simulink library "halout"  (R2021b)
settings: Solver=VariableStepAuto  StartTime=0.0  StopTime=10.0  RelTol=1e-3
undefined symbols (not defined in the file): C_TASK_5MS_S, FALSE, KHAL_CAN1FD1APS3E2E_flg, KHAL_CAN1FD1APS3TxReq_flg, KHAL_CAN1FD1VCU2E2E_flg, KHAL_CAN1FD1VCU2TxReq_flg, KHAL_CAN1FD1VCU3E2E_flg, KHAL_CAN1FD1VCU3TxReq_flg, KHAL_CAN1TxReq_flg, KHAL_CAN1VMCFCM1E2E_flg, KHAL_CAN1VMCFCM1TxReq_flg, KHAL_CAN2TxReq_flg, KHAL_CAN3FD3VCU1toNIDECTxReq_flg, KHAL_CAN3FD3VCU1TxReq_flg, KHAL_CAN3FD3VCU2E2E_flg, KHAL_CAN3FD3VCU2toNIDECE2E_flg, KHAL_CAN3FD3VCU2toNIDECTxReq_flg, KHAL_CAN3FD3VCU2TxReq_flg, KHAL_CAN3TxReq_flg, KHAL_CAN4FD4CE1000E2E_flg, KHAL_CAN4FD4CE1000TxReq_flg, KHAL_CAN4TxReq_flg, KHAL_CAN5TxReq_flg, KHAL_CAN6FD6APS3E2E_flg, KHAL_CAN6FD6APS3TxReq_flg, KHAL_CAN6FD6VCU2E2E_flg, KHAL_CAN6FD6VCU2TxReq_flg, KHAL_CAN6TxReq_flg, ONE_INT, TRUE, ZERO_INT
libraries: FVT_lib x551, simulink x244
(part 25 of 26)

== system halout/HAL_OUT/CAN6/FD6_VCU2_0x154/Byte_11 ==
  VehActPwr : Inport
  BitwiseOR : simulink/Logic and Bit Operations/Bitwise Operator  logicop=OR  UseBitMask=off  BitMask=bin2dec('11011001')  BitMaskRealWorld=Stored Integer
  SignalPack : FVT_lib/hal/SignalPack  RightShiftCnt=8  BitMask=2^8-1  LeftShiftCnt=0
  UnitConverter : DataTypeConversion  OutDataTypeStr=uint8  RndMeth=Round
  UnitConverter1 : DataTypeConversion  OutDataTypeStr=uint32  RndMeth=Round
  convert_out : FVT_lib/hal/convert_out  gain=1  offset=-600000
  Byte_11 : Outport
  wires:
  BitwiseOR/1 -> Byte_11/1
  UnitConverter/1 -> BitwiseOR/1
  SignalPack/1 -> UnitConverter/1
  UnitConverter1/1 -> SignalPack/1
  convert_out/1 -> UnitConverter1/1
  VehActPwr/1 -> convert_out/1

== system halout/HAL_OUT/CAN6/FD6_VCU2_0x154/Byte_12 ==
  VehActPwr : Inport
  BitwiseOR : simulink/Logic and Bit Operations/Bitwise Operator  logicop=OR  UseBitMask=off  BitMask=bin2dec('11011001')  BitMaskRealWorld=Stored Integer
  SignalPack : FVT_lib/hal/SignalPack  RightShiftCnt=0  BitMask=2^8-1  LeftShiftCnt=0
  UnitConverter : DataTypeConversion  OutDataTypeStr=uint8  RndMeth=Round
  UnitConverter1 : DataTypeConversion  OutDataTypeStr=uint32  RndMeth=Round
  convert_out : FVT_lib/hal/convert_out  gain=1  offset=-600000
  Byte_12 : Outport
  wires:
  BitwiseOR/1 -> Byte_12/1
  UnitConverter/1 -> BitwiseOR/1
  SignalPack/1 -> UnitConverter/1
  UnitConverter1/1 -> SignalPack/1
  convert_out/1 -> UnitConverter1/1
  VehActPwr/1 -> convert_out/1

== system halout/HAL_OUT/CAN6/FD6_VCU2_0x154/Byte_13 ==
  DriverTq : Inport
  BitwiseOR : simulink/Logic and Bit Operations/Bitwise Operator  logicop=OR  UseBitMask=off  BitMask=bin2dec('11011001')  BitMaskRealWorld=Stored Integer
  SignalPack : FVT_lib/hal/SignalPack  RightShiftCnt=8  BitMask=2^8-1  LeftShiftCnt=0
  UnitConverter : DataTypeConversion  OutDataTypeStr=uint8  RndMeth=Round
  UnitConverter1 : DataTypeConversion  OutDataTypeStr=uint16  RndMeth=Round
  convert_out : FVT_lib/hal/convert_out  gain=1  offset=-4300
  Byte_13 : Outport
  wires:
  BitwiseOR/1 -> Byte_13/1
  UnitConverter/1 -> BitwiseOR/1
  SignalPack/1 -> UnitConverter/1
  UnitConverter1/1 -> SignalPack/1
  convert_out/1 -> UnitConverter1/1
  DriverTq/1 -> convert_out/1

== system halout/HAL_OUT/CAN6/FD6_VCU2_0x154/Byte_14 ==
  DriverTq : Inport
  BitwiseOR : simulink/Logic and Bit Operations/Bitwise Operator  logicop=OR  UseBitMask=off  BitMask=bin2dec('11011001')  BitMaskRealWorld=Stored Integer
  SignalPack : FVT_lib/hal/SignalPack  RightShiftCnt=0  BitMask=2^8-1  LeftShiftCnt=0
  UnitConverter : DataTypeConversion  OutDataTypeStr=uint8  RndMeth=Round
  UnitConverter1 : DataTypeConversion  OutDataTypeStr=uint16  RndMeth=Round
  convert_out : FVT_lib/hal/convert_out  gain=1  offset=-4300
  Byte_14 : Outport
  wires:
  BitwiseOR/1 -> Byte_14/1
  UnitConverter/1 -> BitwiseOR/1
  SignalPack/1 -> UnitConverter/1
  UnitConverter1/1 -> SignalPack/1
  convert_out/1 -> UnitConverter1/1
  DriverTq/1 -> convert_out/1

== system halout/HAL_OUT/CAN6/FD6_VCU2_0x154/Byte_15 ==
  ActAPSPosn : Inport
  BitwiseOR : simulink/Logic and Bit Operations/Bitwise Operator  logicop=OR  UseBitMask=off  BitMask=bin2dec('11011001')  BitMaskRealWorld=Stored Integer
  SignalPack : FVT_lib/hal/SignalPack  RightShiftCnt=0  BitMask=2^8-1  LeftShiftCnt=0
  UnitConverter : DataTypeConversion  OutDataTypeStr=uint8  RndMeth=Round
  UnitConverter1 : DataTypeConversion  OutDataTypeStr=uint8  RndMeth=Round
  convert_out : FVT_lib/hal/convert_out  gain=0.394  offset=0
  Byte_15 : Outport
  wires:
  BitwiseOR/1 -> Byte_15/1
  UnitConverter/1 -> BitwiseOR/1
  SignalPack/1 -> UnitConverter/1
  UnitConverter1/1 -> SignalPack/1
  convert_out/1 -> UnitConverter1/1
  ActAPSPosn/1 -> convert_out/1

== system halout/HAL_OUT/CAN6/FD6_VCU2_0x154/Byte_2 ==
  Fr_DriverTq : Inport
  BitwiseOR : simulink/Logic and Bit Operations/Bitwise Operator  logicop=OR  UseBitMask=off  BitMask=bin2dec('11011001')  BitMaskRealWorld=Stored Integer
  SignalPack : FVT_lib/hal/SignalPack  RightShiftCnt=8  BitMask=2^8-1  LeftShiftCnt=0
  UnitConverter : DataTypeConversion  OutDataTypeStr=uint8  RndMeth=Round
  UnitConverter1 : DataTypeConversion  OutDataTypeStr=uint16  RndMeth=Round
  convert_out : FVT_lib/hal/convert_out  gain=0.5  offset=-5300
  Byte_2 : Outport
  wires:
  BitwiseOR/1 -> Byte_2/1
  UnitConverter/1 -> BitwiseOR/1
  SignalPack/1 -> UnitConverter/1
  UnitConverter1/1 -> SignalPack/1
  convert_out/1 -> UnitConverter1/1
  Fr_DriverTq/1 -> convert_out/1

== system halout/HAL_OUT/CAN6/FD6_VCU2_0x154/Byte_3 ==
  Fr_DriverTq : Inport
  BitwiseOR : simulink/Logic and Bit Operations/Bitwise Operator  logicop=OR  UseBitMask=off  BitMask=bin2dec('11011001')  BitMaskRealWorld=Stored Integer
  SignalPack : FVT_lib/hal/SignalPack  RightShiftCnt=0  BitMask=2^8-1  LeftShiftCnt=0
  UnitConverter : DataTypeConversion  OutDataTypeStr=uint8  RndMeth=Round
  UnitConverter1 : DataTypeConversion  OutDataTypeStr=uint16  RndMeth=Round
  convert_out : FVT_lib/hal/convert_out  gain=0.5  offset=-5300
  Byte_3 : Outport
  wires:
  BitwiseOR/1 -> Byte_3/1
  UnitConverter/1 -> BitwiseOR/1
  SignalPack/1 -> UnitConverter/1
  UnitConverter1/1 -> SignalPack/1
  convert_out/1 -> UnitConverter1/1
  Fr_DriverTq/1 -> convert_out/1

== system halout/HAL_OUT/CAN6/FD6_VCU2_0x154/Byte_4 ==
  Rr_DriverTq : Inport
  BitwiseOR : simulink/Logic and Bit Operations/Bitwise Operator  logicop=OR  UseBitMask=off  BitMask=bin2dec('11011001')  BitMaskRealWorld=Stored Integer
  SignalPack : FVT_lib/hal/SignalPack  RightShiftCnt=8  BitMask=2^8-1  LeftShiftCnt=0
  UnitConverter : DataTypeConversion  OutDataTypeStr=uint8  RndMeth=Round
  UnitConverter1 : DataTypeConversion  OutDataTypeStr=uint16  RndMeth=Round
  convert_out : FVT_lib/hal/convert_out  gain=0.5  offset=-5300
  Byte_4 : Outport
  wires:
  BitwiseOR/1 -> Byte_4/1
  UnitConverter/1 -> BitwiseOR/1
  SignalPack/1 -> UnitConverter/1
  UnitConverter1/1 -> SignalPack/1
  convert_out/1 -> UnitConverter1/1
  Rr_DriverTq/1 -> convert_out/1

== system halout/HAL_OUT/CAN6/FD6_VCU2_0x154/Byte_5 ==
  Rr_DriverTq : Inport
  BitwiseOR : simulink/Logic and Bit Operations/Bitwise Operator  logicop=OR  UseBitMask=off  BitMask=bin2dec('11011001')  BitMaskRealWorld=Stored Integer
  SignalPack : FVT_lib/hal/SignalPack  RightShiftCnt=0  BitMask=2^8-1  LeftShiftCnt=0
  UnitConverter : DataTypeConversion  OutDataTypeStr=uint8  RndMeth=Round
  UnitConverter1 : DataTypeConversion  OutDataTypeStr=uint16  RndMeth=Round
  convert_out : FVT_lib/hal/convert_out  gain=0.5  offset=-5300
  Byte_5 : Outport
  wires:
  BitwiseOR/1 -> Byte_5/1
  UnitConverter/1 -> BitwiseOR/1
  SignalPack/1 -> UnitConverter/1
  UnitConverter1/1 -> SignalPack/1
  convert_out/1 -> UnitConverter1/1
  Rr_DriverTq/1 -> convert_out/1

== system halout/HAL_OUT/CAN6/FD6_VCU2_0x154/Byte_6 ==
  ACC_CtrlAvail : Inport
  AccPedal_Override : Inport  Port=2
  BitwiseOR : simulink/Logic and Bit Operations/Bitwise Operator  logicop=OR  UseBitMask=off  NumInputPorts=2  BitMask=bin2dec('11011001')  BitMaskRealWorld=Stored Integer
  SignalPack : FVT_lib/hal/SignalPack  RightShiftCnt=0  BitMask=2^1-1  LeftShiftCnt=7
  SignalPack1 : FVT_lib/hal/SignalPack  RightShiftCnt=0  BitMask=2^1-1  LeftShiftCnt=6
  UnitConverter{,1..3} (4 alike) : DataTypeConversion  OutDataTypeStr=uint8  RndMeth=Round
  Byte_6 : Outport
  wires:
  BitwiseOR/1 -> Byte_6/1
  UnitConverter/1 -> BitwiseOR/1
  SignalPack/1 -> UnitConverter/1
  UnitConverter1/1 -> SignalPack/1
  ACC_CtrlAvail/1 -> UnitConverter1/1
  UnitConverter2/1 -> BitwiseOR/2
  SignalPack1/1 -> UnitConverter2/1
  UnitConverter3/1 -> SignalPack1/1
  AccPedal_Override/1 -> UnitConverter3/1

== system halout/HAL_OUT/CAN6/FD6_VCU2_0x154/CRC8_IfAction_Tx ==
  CAN_E2E_flg : Inport
  DataID1 : Inport  Port=2
  DataID2 : Inport  Port=3
  RawData : Inport  Port=4
  Data Type Conversion : DataTypeConversion  OutDataTypeStr=uint8
  If : If
  If Action Subsystem : Subsystem  TreatAsAtomicUnit=on
  If Action Subsystem1 : Subsystem  TreatAsAtomicUnit=on
  Merge : Merge
  CRC8 : Outport
  wires:
  If/2 -> If Action Subsystem/Action
  If/1 -> If Action Subsystem1/Action
  CAN_E2E_flg/1 -> [CAN_E2E_flg]
  DataID1/1 -> [DataID1]
  DataID2/1 -> [DataID2]
  RawData/1 -> [RawData]
  [CAN_E2E_flg] -> Data Type Conversion/1
  [DataID1] -> If Action Subsystem1/1(CAN_E2E_ID1)
  [DataID2] -> If Action Subsystem1/2(CAN_E2E_ID2)
  [RawData] -> If Action Subsystem1/3(Byte1)
  [RawData] -> If Action Subsystem/1(Byte1)
  If Action Subsystem1/1(CRC8_E2EResult) -> Merge/1
  If Action Subsystem/1(CRC8_Result) -> Merge/2
  Merge/1 -> CRC8/1
  Data Type Conversion/1 -> If/1

== system halout/HAL_OUT/CAN6/FD6_VCU2_0x154/CSVCU2CAN6 ==
  CSVCU2CAN6 : Inport
  Data Type Conversion : DataTypeConversion  OutDataTypeStr=uint8  RndMeth=Round
  CAN6_CS_VCU2_CAN6 : Outport
  wires:
  Data Type Conversion/1 -> CAN6_CS_VCU2_CAN6/1
  CSVCU2CAN6/1 -> Data Type Conversion/1

== system halout/HAL_OUT/CAN6/FD6_VCU2_0x154/DriverTq ==
  DriverTq : Inport
  Data Type Conversion : DataTypeConversion  OutDataTypeStr=uint16  RndMeth=Round
  convert_out : FVT_lib/hal/convert_out  gain=1  offset=-4300
  CAN6_DriverTq : Outport
  wires:
  Data Type Conversion/1 -> CAN6_DriverTq/1
  convert_out/1 -> Data Type Conversion/1
  DriverTq/1 -> convert_out/1

== system halout/HAL_OUT/CAN6/FD6_VCU2_0x154/FrDriverTq ==
  FrDriverTq : Inport
  Data Type Conversion : DataTypeConversion  OutDataTypeStr=uint16  RndMeth=Round
  convert_out : FVT_lib/hal/convert_out  gain=0.5  offset=-5300
  CAN6_Fr_DriverTq : Outport
  wires:
  Data Type Conversion/1 -> CAN6_Fr_DriverTq/1
  convert_out/1 -> Data Type Conversion/1
  FrDriverTq/1 -> convert_out/1

== system halout/HAL_OUT/CAN6/FD6_VCU2_0x154/RCVCU2CAN6 ==
  RCVCU2CAN6 : Inport
  Data Type Conversion : DataTypeConversion  OutDataTypeStr=uint8  RndMeth=Round
  CAN6_RC_VCU2_CAN6 : Outport
  wires:
  Data Type Conversion/1 -> CAN6_RC_VCU2_CAN6/1
  RCVCU2CAN6/1 -> Data Type Conversion/1

== system halout/HAL_OUT/CAN6/FD6_VCU2_0x154/RrDriverTq ==
  RrDriverTq : Inport
  Data Type Conversion : DataTypeConversion  OutDataTypeStr=uint16  RndMeth=Round
  convert_out : FVT_lib/hal/convert_out  gain=0.5  offset=-5300
  CAN6_Rr_DriverTq : Outport
  wires:
  Data Type Conversion/1 -> CAN6_Rr_DriverTq/1
  convert_out/1 -> Data Type Conversion/1
  RrDriverTq/1 -> convert_out/1

== system halout/HAL_OUT/CAN6/FD6_VCU2_0x154/VehActPwr ==
  VehActPwr : Inport
  Data Type Conversion : DataTypeConversion  OutDataTypeStr=uint32  RndMeth=Round
  convert_out : FVT_lib/hal/convert_out  gain=1  offset=-600000
  CAN6_VehActPwr : Outport
  wires:
  Data Type Conversion/1 -> CAN6_VehActPwr/1
  convert_out/1 -> Data Type Conversion/1
  VehActPwr/1 -> convert_out/1

== system halout/HAL_OUT/CAN6/FD6_VMC1_0x17F/AccCalcuPID ==
  AccCalcuPID : Inport
  Data Type Conversion : DataTypeConversion  OutDataTypeStr=uint16  RndMeth=Round
  convert_out : FVT_lib/hal/convert_out  gain=0.05  offset=-15
  CAN6_AccCalcuPID : Outport
  wires:
  Data Type Conversion/1 -> CAN6_AccCalcuPID/1
  convert_out/1 -> Data Type Conversion/1
  AccCalcuPID/1 -> convert_out/1

== system halout/HAL_OUT/CAN6/FD6_VMC1_0x17F/CCMSASpdWar ==
  CCMSASpdWar : Inport
  Data Type Conversion : DataTypeConversion  OutDataTypeStr=uint8  RndMeth=Round
  CAN6_CCMSA_SpdWar : Outport
  wires:
  Data Type Conversion/1 -> CAN6_CCMSA_SpdWar/1
  CCMSASpdWar/1 -> Data Type Conversion/1

== system halout/HAL_OUT/CAN6/FD6_VMC1_0x17F/DISCButtSta ==
  DISCButtSta : Inport
  Data Type Conversion : DataTypeConversion  OutDataTypeStr=uint8  RndMeth=Round
  CAN6_DISC_ButtSta : Outport
  wires:
  Data Type Conversion/1 -> CAN6_DISC_ButtSta/1
  DISCButtSta/1 -> Data Type Conversion/1

== system halout/HAL_OUT/CAN6/FD6_VMC1_0x17F/DISCDISCTargetSpd ==
  DISCDISCTargetSpd : Inport
  Data Type Conversion : DataTypeConversion  OutDataTypeStr=uint16  RndMeth=Round
  convert_out : FVT_lib/hal/convert_out  gain=0.125  offset=0
  CAN6_DISC_DISCTargetSpd : Outport
  wires:
  Data Type Conversion/1 -> CAN6_DISC_DISCTargetSpd/1
  convert_out/1 -> Data Type Conversion/1
  DISCDISCTargetSpd/1 -> convert_out/1

== system halout/HAL_OUT/CAN6/FD6_VMC1_0x17F/DISCDISCTurn ==
  DISCDISCTurn : Inport
  Data Type Conversion : DataTypeConversion  OutDataTypeStr=uint8  RndMeth=Round
  CAN6_DISC_DISCTurn : Outport
  wires:
  Data Type Conversion/1 -> CAN6_DISC_DISCTurn/1
  DISCDISCTurn/1 -> Data Type Conversion/1

== system halout/HAL_OUT/CAN6/FD6_VMC1_0x17F/DISCReqAcc ==
  DISCReqAcc : Inport
  Data Type Conversion : DataTypeConversion  OutDataTypeStr=uint16  RndMeth=Round
  convert_out : FVT_lib/hal/convert_out  gain=0.05  offset=-15
  CAN6_DISCReqAcc : Outport
  wires:
  Data Type Conversion/1 -> CAN6_DISCReqAcc/1
  convert_out/1 -> Data Type Conversion/1
  DISCReqAcc/1 -> convert_out/1

== system halout/HAL_OUT/CAN6/FD6_VMC1_0x17F/DISCSta ==
  DISCSta : Inport
  Data Type Conversion : DataTypeConversion  OutDataTypeStr=uint8  RndMeth=Round
  CAN6_DISC_Sta : Outport
  wires:
  Data Type Conversion/1 -> CAN6_DISC_Sta/1
  DISCSta/1 -> Data Type Conversion/1

== system halout/HAL_OUT/CAN6/FD6_VMC1_0x17F/FDCVMCLongAccelCmd ==
  FDCVMCLongAccelCmd : Inport
  Data Type Conversion : DataTypeConversion  OutDataTypeStr=uint8  RndMeth=Round
  convert_out : FVT_lib/hal/convert_out  gain=0.01  offset=-1.27
  CAN6_FDC_VMC_LongAccel_Cmd : Outport
  wires:
  Data Type Conversion/1 -> CAN6_FDC_VMC_LongAccel_Cmd/1
  convert_out/1 -> Data Type Conversion/1
  FDCVMCLongAccelCmd/1 -> convert_out/1

== system halout/HAL_OUT/CAN6/FD6_VMC1_0x17F/FeatArbitrFinal ==
  FeatArbitrFinal : Inport
  Data Type Conversion : DataTypeConversion  OutDataTypeStr=uint8  RndMeth=Round
  CAN6_FeatArbitrFinal : Outport
  wires:
  Data Type Conversion/1 -> CAN6_FeatArbitrFinal/1
  FeatArbitrFinal/1 -> Data Type Conversion/1

== system halout/HAL_OUT/CAN6/FD6_VMC1_0x17F/FeatArbitrSta ==
  FeatArbitrSta : Inport
  Data Type Conversion : DataTypeConversion  OutDataTypeStr=uint8  RndMeth=Round
  CAN6_FeatArbitrSta : Outport
  wires:
  Data Type Conversion/1 -> CAN6_FeatArbitrSta/1
  FeatArbitrSta/1 -> Data Type Conversion/1

== system halout/HAL_OUT/CAN6/FD6_VMC1_0x17F/FeatReqSpd ==
  FeatReqSpd : Inport
  Data Type Conversion : DataTypeConversion  OutDataTypeStr=uint16  RndMeth=Round
  convert_out : FVT_lib/hal/convert_out  gain=0.125  offset=0
  CAN6_FeatReqSpd : Outport
  wires:
  Data Type Conversion/1 -> CAN6_FeatReqSpd/1
  convert_out/1 -> Data Type Conversion/1
  FeatReqSpd/1 -> convert_out/1

== system halout/HAL_OUT/CAN6/FD6_VMC1_0x17F/FeatSetSpdFinalraw32 ==
  FeatSetSpdFinalraw32 : Inport
  Data Type Conversion : DataTypeConversion  OutDataTypeStr=uint8  RndMeth=Round
  CAN6_FeatSetSpdFinal_raw32 : Outport
  wires:
  Data Type Conversion/1 -> CAN6_FeatSetSpdFinal_raw32/1
  FeatSetSpdFinalraw32/1 -> Data Type Conversion/1

== system halout/HAL_OUT/CAN6/FD6_VMC1_0x17F/FrontRearSlipRatioCtrl ==
  FrontRearSlipRatioCtrl : Inport
  Data Type Conversion : DataTypeConversion  OutDataTypeStr=uint8  RndMeth=Round
  CAN6_FrontRearSlipRatioCtrl : Outport
  wires:
  Data Type Conversion/1 -> CAN6_FrontRearSlipRatioCtrl/1
  FrontRearSlipRatioCtrl/1 -> Data Type Conversion/1

== system halout/HAL_OUT/CAN6/FD6_VMC1_0x17F/JerkPCT ==
  JerkPCT : Inport
  Data Type Conversion : DataTypeConversion  OutDataTypeStr=uint8  RndMeth=Round
  CAN6_JerkPCT : Outport
  wires:
  Data Type Conversion/1 -> CAN6_JerkPCT/1
  JerkPCT/1 -> Data Type Conversion/1

== system halout/HAL_OUT/CAN6/FD6_VMC1_0x17F/LatAccCtrl ==
  LatAccCtrl : Inport
  Data Type Conversion : DataTypeConversion  OutDataTypeStr=uint8  RndMeth=Round
  CAN6_LatAccCtrl : Outport
  wires:
  Data Type Conversion/1 -> CAN6_LatAccCtrl/1
  LatAccCtrl/1 -> Data Type Conversion/1

== system halout/HAL_OUT/CAN6/FD6_VMC1_0x17F/LateralCtrl ==
  LateralCtrl : Inport
  Data Type Conversion : DataTypeConversion  OutDataTypeStr=uint8  RndMeth=Round
  CAN6_LateralCtrl : Outport
  wires:
  Data Type Conversion/1 -> CAN6_LateralCtrl/1
  LateralCtrl/1 -> Data Type Conversion/1

== system halout/HAL_OUT/CAN6/FD6_VMC1_0x17F/LimitPCT ==
  LimitPCT : Inport
  Data Type Conversion : DataTypeConversion  OutDataTypeStr=uint8  RndMeth=Round
  CAN6_LimitPCT : Outport
  wires:
  Data Type Conversion/1 -> CAN6_LimitPCT/1
  LimitPCT/1 -> Data Type Conversion/1

== system halout/HAL_OUT/CAN6/FD6_VMC1_0x17F/MeterIndSpeedraw32 ==
  MeterIndSpeedraw32 : Inport
  Data Type Conversion : DataTypeConversion  OutDataTypeStr=uint8  RndMeth=Round
  CAN6_MeterIndSpeed_raw32 : Outport
  wires:
  Data Type Conversion/1 -> CAN6_MeterIndSpeed_raw32/1
  MeterIndSpeedraw32/1 -> Data Type Conversion/1

== system halout/HAL_OUT/CAN6/FD6_VMC1_0x17F/RearWhlSlipRatioCtrl ==
  RearWhlSlipRatioCtrl : Inport
  Data Type Conversion : DataTypeConversion  OutDataTypeStr=uint8  RndMeth=Round
  CAN6_RearWhlSlipRatioCtrl : Outport
  wires:
  Data Type Conversion/1 -> CAN6_RearWhlSlipRatioCtrl/1
  RearWhlSlipRatioCtrl/1 -> Data Type Conversion/1

== system halout/HAL_OUT/CAN6/FD6_VMC1_0x17F/SPD2ACCAct ==
  SPD2ACCAct : Inport
  Data Type Conversion : DataTypeConversion  OutDataTypeStr=uint8  RndMeth=Round
  CAN6_SPD2ACCAct : Outport
  wires:
  Data Type Conversion/1 -> CAN6_SPD2ACCAct/1
  SPD2ACCAct/1 -> Data Type Conversion/1

== system halout/HAL_OUT/CAN6/FD6_VMC1_0x17F/SafetyCtrl ==
  SafetyCtrl : Inport
  Data Type Conversion : DataTypeConversion  OutDataTypeStr=uint8  RndMeth=Round
  CAN6_SafetyCtrl : Outport
  wires:
  Data Type Conversion/1 -> CAN6_SafetyCtrl/1
  SafetyCtrl/1 -> Data Type Conversion/1

== system halout/HAL_OUT/CAN6/FD6_VMC1_0x17F/SingleWhlSlipRatioCtrl ==
  SingleWhlSlipRatioCtrl : Inport
  Data Type Conversion : DataTypeConversion  OutDataTypeStr=uint8  RndMeth=Round
  CAN6_SingleWhlSlipRatioCtrl : Outport
  wires:
  Data Type Conversion/1 -> CAN6_SingleWhlSlipRatioCtrl/1
  SingleWhlSlipRatioCtrl/1 -> Data Type Conversion/1

== system halout/HAL_OUT/CAN6/FD6_VMC1_0x17F/TimeGapCalcu ==
  TimeGapCalcu : Inport
  Data Type Conversion : DataTypeConversion  OutDataTypeStr=uint8  RndMeth=Round
  convert_out : FVT_lib/hal/convert_out  gain=0.1  offset=0
  CAN6_TimeGapCalcu : Outport
  wires:
  Data Type Conversion/1 -> CAN6_TimeGapCalcu/1
  convert_out/1 -> Data Type Conversion/1
  TimeGapCalcu/1 -> convert_out/1

== system halout/HAL_OUT/CAN6/FD6_VMC1_0x17F/VMCACCCtrlAvail ==
  VMCACCCtrlAvail : Inport
  Data Type Conversion : DataTypeConversion  OutDataTypeStr=uint8  RndMeth=Round
  CAN6_VMC_ACCCtrlAvail : Outport
  wires:
  Data Type Conversion/1 -> CAN6_VMC_ACCCtrlAvail/1
  VMCACCCtrlAvail/1 -> Data Type Conversion/1

== system halout/HAL_OUT/CAN6/FD6_VMC1_0x17F/VMCAEBCtrlAvail ==
  VMCAEBCtrlAvail : Inport
  Data Type Conversion : DataTypeConversion  OutDataTypeStr=uint8  RndMeth=Round
  CAN6_VMC_AEBCtrlAvail : Outport
  wires:
  Data Type Conversion/1 -> CAN6_VMC_AEBCtrlAvail/1
  VMCAEBCtrlAvail/1 -> Data Type Conversion/1

== system halout/HAL_OUT/CAN6/FD6_VMC1_0x17F/VMCCCCtrlAvail ==
  VMCCCCtrlAvail : Inport
  Data Type Conversion : DataTypeConversion  OutDataTypeStr=uint8  RndMeth=Round
  CAN6_VMC_CCCtrlAvail : Outport
  wires:
  Data Type Conversion/1 -> CAN6_VMC_CCCtrlAvail/1
  VMCCCCtrlAvail/1 -> Data Type Conversion/1

== system halout/HAL_OUT/CAN6/FD6_VMC1_0x17F/VMCMSACtrlAvail ==
  VMCMSACtrlAvail : Inport
  Data Type Conversion : DataTypeConversion  OutDataTypeStr=uint8  RndMeth=Round
  CAN6_VMC_MSACtrlAvail : Outport
  wires:
  Data Type Conversion/1 -> CAN6_VMC_MSACtrlAvail/1
  VMCMSACtrlAvail/1 -> Data Type Conversion/1

== system halout/HAL_OUT/CAN6/FD6_VMC1_0x17F/VMCVCUACCCtrlAvail ==
  VMCVCUACCCtrlAvail : Inport
  Data Type Conversion : DataTypeConversion  OutDataTypeStr=uint8  RndMeth=Round
  CAN6_VMC_VCU_ACC_CtrlAvail : Outport
  wires:
  Data Type Conversion/1 -> CAN6_VMC_VCU_ACC_CtrlAvail/1
  VMCVCUACCCtrlAvail/1 -> Data Type Conversion/1

== system halout/HAL_OUT/CAN6/FD6_VMC1_0x17F/VMCVCUAPSCtrlAvailflg ==
  VMCVCUAPSCtrlAvailflg : Inport
  Data Type Conversion : DataTypeConversion  OutDataTypeStr=uint8  RndMeth=Round
  CAN6_VMC_VCU_APSCtrlAvail_flg : Outport
  wires:
  Data Type Conversion/1 -> CAN6_VMC_VCU_APSCtrlAvail_flg/1
  VMCVCUAPSCtrlAvailflg/1 -> Data Type Conversion/1

== system halout/HAL_OUT/CAN6/FD6_VMC1_0x17F/VMCVCUAccPedalOverride ==
  VMCVCUAccPedalOverride : Inport
  Data Type Conversion : DataTypeConversion  OutDataTypeStr=uint8  RndMeth=Round
  CAN6_VMC_VCU_AccPedal_Override : Outport
  wires:
  Data Type Conversion/1 -> CAN6_VMC_VCU_AccPedal_Override/1
  VMCVCUAccPedalOverride/1 -> Data Type Conversion/1

== system halout/HAL_OUT/CAN6/FD6_VMC1_0x17F/VMCVCUCCCrlSta ==
  VMCVCUCCCrlSta : Inport
  Data Type Conversion : DataTypeConversion  OutDataTypeStr=uint8  RndMeth=Round
  CAN6_VMC_VCU_CC_Crl_Sta : Outport
  wires:
  Data Type Conversion/1 -> CAN6_VMC_VCU_CC_Crl_Sta/1
  VMCVCUCCCrlSta/1 -> Data Type Conversion/1

== system halout/HAL_OUT/CAN6/FD6_VMC1_0x17F/VMCVCUMSACrlSta ==
  VMCVCUMSACrlSta : Inport
  Data Type Conversion : DataTypeConversion  OutDataTypeStr=uint8  RndMeth=Round
  CAN6_VMC_VCU_MSA_Crl_Sta : Outport
  wires:
  Data Type Conversion/1 -> CAN6_VMC_VCU_MSA_Crl_Sta/1
  VMCVCUMSACrlSta/1 -> Data Type Conversion/1

== system halout/HAL_OUT/CAN6/FD6_VMC1_0x17F/VehicleSpeedkph ==
  VehicleSpeedkph : Inport
  Data Type Conversion : DataTypeConversion  OutDataTypeStr=uint16  RndMeth=Round
  convert_out : FVT_lib/hal/convert_out  gain=0.125  offset=0
  CAN6_VehicleSpeed_kph : Outport
  wires:
  Data Type Conversion/1 -> CAN6_VehicleSpeed_kph/1
  convert_out/1 -> Data Type Conversion/1
  VehicleSpeedkph/1 -> convert_out/1

== system halout/HAL_OUT/CAN6/FD6_VMC1_0x17F/VehicleSpeedmph ==
  VehicleSpeedmph : Inport
  Data Type Conversion : DataTypeConversion  OutDataTypeStr=uint16  RndMeth=Round
  convert_out : FVT_lib/hal/convert_out  gain=0.125  offset=0
  CAN6_VehicleSpeed_mph : Outport
  wires:
  Data Type Conversion/1 -> CAN6_VehicleSpeed_mph/1
  convert_out/1 -> Data Type Conversion/1
  VehicleSpeedmph/1 -> convert_out/1

== system halout/HAL_OUT/CAN6/GW6_CE100_0_0x1C6/FDCBCMDimSw ==
  FDCBCMDimSw : Inport
  Data Type Conversion : DataTypeConversion  OutDataTypeStr=uint8  RndMeth=Round
  CAN6_FDC_BCM_DimSw : Outport
  wires:
  Data Type Conversion/1 -> CAN6_FDC_BCM_DimSw/1
  FDCBCMDimSw/1 -> Data Type Conversion/1

== system halout/HAL_OUT/CAN6/GW6_CE100_0_0x1C6/FDCBCMFWipSwSta ==
  FDCBCMFWipSwSta : Inport
  Data Type Conversion : DataTypeConversion  OutDataTypeStr=uint8  RndMeth=Round
  CAN6_FDC_BCM_FWipSw_Sta : Outport
  wires:
  Data Type Conversion/1 -> CAN6_FDC_BCM_FWipSw_Sta/1
  FDCBCMFWipSwSta/1 -> Data Type Conversion/1

== system halout/HAL_OUT/CAN6/GW6_CE100_0_0x1C6/FDCBCMLLeftStaCmd ==
  FDCBCMLLeftStaCmd : Inport
  Data Type Conversion : DataTypeConversion  OutDataTypeStr=uint8  RndMeth=Round
  CAN6_FDC_BCM_LLeftSta_Cmd : Outport
  wires:
  Data Type Conversion/1 -> CAN6_FDC_BCM_LLeftSta_Cmd/1
  FDCBCMLLeftStaCmd/1 -> Data Type Conversion/1

== system halout/HAL_OUT/CAN6/GW6_CE100_0_0x1C6/FDCBCMLRightStaCmd ==
  FDCBCMLRightStaCmd : Inport
  Data Type Conversion : DataTypeConversion  OutDataTypeStr=uint8  RndMeth=Round
  CAN6_FDC_BCM_LRightSta_Cmd : Outport
  wires:
  Data Type Conversion/1 -> CAN6_FDC_BCM_LRightSta_Cmd/1
  FDCBCMLRightStaCmd/1 -> Data Type Conversion/1

== system halout/HAL_OUT/CAN6/GW6_CE100_0_0x1C6/FDCBCMPassSWSta ==
  FDCBCMPassSWSta : Inport
  Data Type Conversion : DataTypeConversion  OutDataTypeStr=uint8  RndMeth=Round
  CAN6_FDC_BCM_PassSW_Sta : Outport
  wires:
  Data Type Conversion/1 -> CAN6_FDC_BCM_PassSW_Sta/1
  FDCBCMPassSWSta/1 -> Data Type Conversion/1

== system halout/HAL_OUT/CAN6/GW6_CE100_0_0x1C6/FDCBCMTurnSwSta ==
  FDCBCMTurnSwSta : Inport
  Data Type Conversion : DataTypeConversion  OutDataTypeStr=uint8  RndMeth=Round
  CAN6_FDC_BCM_TurnSw_Sta : Outport
  wires:
  Data Type Conversion/1 -> CAN6_FDC_BCM_TurnSw_Sta/1
  FDCBCMTurnSwSta/1 -> Data Type Conversion/1

== system halout/HAL_OUT/CAN6/GW6_CE100_0_0x1C6/FDCVMCSpdCtrlModeSta ==
  FDCVMCSpdCtrlModeSta : Inport
  Data Type Conversion : DataTypeConversion  OutDataTypeStr=uint8  RndMeth=Round
  CAN6_FDC_VMC_SpdCtrlMode_Sta : Outport
  wires:
  Data Type Conversion/1 -> CAN6_FDC_VMC_SpdCtrlMode_Sta/1
  FDCVMCSpdCtrlModeSta/1 -> Data Type Conversion/1

== system halout/HAL_OUT/CAN6/GW6_CE100_0_0x1C6/FDCVMCSpdCtrlSta ==
  FDCVMCSpdCtrlSta : Inport
  Data Type Conversion : DataTypeConversion  OutDataTypeStr=uint8  RndMeth=Round
  CAN6_FDC_VMC_SpdCtrl_Sta : Outport
  wires:
  Data Type Conversion/1 -> CAN6_FDC_VMC_SpdCtrl_Sta/1
  FDCVMCSpdCtrlSta/1 -> Data Type Conversion/1

== system halout/HAL_OUT/CAN1/FD1_APS3_0x238/CRC8_IfAction_Tx/If Action Subsystem ==
  Byte1 : Inport
  Action Port : ActionPort
  CRC8_Caculation : Subsystem
      mask help: MeasumentTrigerEvent
      mask Display: fprintf('CRC8');
  CRC8_Result : Outport
  wires:
  CRC8_Caculation/1(CRCout) -> CRC8_Result/1
  Byte1/1 -> CRC8_Caculation/1(MsgData)

== system halout/HAL_OUT/CAN1/FD1_APS3_0x238/CRC8_IfAction_Tx/If Action Subsystem1 ==
  CAN_E2E_ID1 : Inport
  CAN_E2E_ID2 : Inport  Port=2
  Byte1 : Inport  Port=3
  Action Port : ActionPort
  CRC8_E2EProfile1 : Subsystem
      mask help: MeasumentTrigerEvent
      mask Display: fprintf('CRC8_E2EProfile1');
  Mux2 : Mux  Inputs=3
  CRC8_E2EResult : Outport
  wires:
  Mux2/1 -> CRC8_E2EProfile1/1(MsgData)
  CAN_E2E_ID1/1 -> Mux2/1
  CAN_E2E_ID2/1 -> Mux2/2
  Byte1/1 -> Mux2/3
  CRC8_E2EProfile1/1(CRCout) -> CRC8_E2EResult/1

== system halout/HAL_OUT/CAN1/FD1_VCU2_0x154/CRC8_IfAction_Tx/If Action Subsystem ==
  Byte1 : Inport
  Action Port : ActionPort
  CRC8_Caculation : Subsystem
      mask help: MeasumentTrigerEvent
      mask Display: fprintf('CRC8');
  CRC8_Result : Outport
  wires:
  CRC8_Caculation/1(CRCout) -> CRC8_Result/1
  Byte1/1 -> CRC8_Caculation/1(MsgData)

== system halout/HAL_OUT/CAN1/FD1_VCU2_0x154/CRC8_IfAction_Tx/If Action Subsystem1 ==
  CAN_E2E_ID1 : Inport
  CAN_E2E_ID2 : Inport  Port=2
  Byte1 : Inport  Port=3
  Action Port : ActionPort
  CRC8_E2EProfile1 : Subsystem
      mask help: MeasumentTrigerEvent
      mask Display: fprintf('CRC8_E2EProfile1');
  Mux2 : Mux  Inputs=3
  CRC8_E2EResult : Outport
  wires:
  Mux2/1 -> CRC8_E2EProfile1/1(MsgData)
  CAN_E2E_ID1/1 -> Mux2/1
  CAN_E2E_ID2/1 -> Mux2/2
  Byte1/1 -> Mux2/3
  CRC8_E2EProfile1/1(CRCout) -> CRC8_E2EResult/1

== system halout/HAL_OUT/CAN1/FD1_VCU3_0x159/CRC8_IfAction_Tx/If Action Subsystem ==
  Byte1 : Inport
  Action Port : ActionPort
  CRC8_Caculation : Subsystem
      mask help: MeasumentTrigerEvent
      mask Display: fprintf('CRC8');
  CRC8_Result : Outport
  wires:
  CRC8_Caculation/1(CRCout) -> CRC8_Result/1
  Byte1/1 -> CRC8_Caculation/1(MsgData)

== system halout/HAL_OUT/CAN1/FD1_VCU3_0x159/CRC8_IfAction_Tx/If Action Subsystem1 ==
  CAN_E2E_ID1 : Inport
  CAN_E2E_ID2 : Inport  Port=2
  Byte1 : Inport  Port=3
  Action Port : ActionPort
  CRC8_E2EProfile1 : Subsystem
      mask help: MeasumentTrigerEvent
      mask Display: fprintf('CRC8_E2EProfile1');
  Mux2 : Mux  Inputs=3
  CRC8_E2EResult : Outport
  wires:
  Mux2/1 -> CRC8_E2EProfile1/1(MsgData)
  CAN_E2E_ID1/1 -> Mux2/1
  CAN_E2E_ID2/1 -> Mux2/2
  Byte1/1 -> Mux2/3
  CRC8_E2EProfile1/1(CRCout) -> CRC8_E2EResult/1

== system halout/HAL_OUT/CAN1/VMC_FCM1_0x172/CRC8_IfAction_Tx/If Action Subsystem ==
  Byte1 : Inport
  Action Port : ActionPort
  CRC8_Caculation : Subsystem
      mask help: MeasumentTrigerEvent
      mask Display: fprintf('CRC8');
  CRC8_Result : Outport
  wires:
  CRC8_Caculation/1(CRCout) -> CRC8_Result/1
  Byte1/1 -> CRC8_Caculation/1(MsgData)

== system halout/HAL_OUT/CAN1/VMC_FCM1_0x172/CRC8_IfAction_Tx/If Action Subsystem1 ==
  CAN_E2E_ID1 : Inport
  CAN_E2E_ID2 : Inport  Port=2
  Byte1 : Inport  Port=3
  Action Port : ActionPort
  CRC8_E2EProfile1 : Subsystem
      mask help: MeasumentTrigerEvent
      mask Display: fprintf('CRC8_E2EProfile1');
  Mux2 : Mux  Inputs=3
  CRC8_E2EResult : Outport
  wires:
  Mux2/1 -> CRC8_E2EProfile1/1(MsgData)
  CAN_E2E_ID1/1 -> Mux2/1
  CAN_E2E_ID2/1 -> Mux2/2
  Byte1/1 -> Mux2/3
  CRC8_E2EProfile1/1(CRCout) -> CRC8_E2EResult/1

== system halout/HAL_OUT/CAN3/FD3_VCU2_0x153/CRC8_IfAction_Tx/If Action Subsystem ==
  Byte1 : Inport
  Action Port : ActionPort
  CRC8_Caculation : Subsystem
      mask help: MeasumentTrigerEvent
      mask Display: fprintf('CRC8');
  CRC8_Result : Outport
  wires:
  CRC8_Caculation/1(CRCout) -> CRC8_Result/1
  Byte1/1 -> CRC8_Caculation/1(MsgData)

== system halout/HAL_OUT/CAN3/FD3_VCU2_0x153/CRC8_IfAction_Tx/If Action Subsystem1 ==
  CAN_E2E_ID1 : Inport
  CAN_E2E_ID2 : Inport  Port=2
  Byte1 : Inport  Port=3
  Action Port : ActionPort
  CRC8_E2EProfile1 : Subsystem
      mask help: MeasumentTrigerEvent
      mask Display: fprintf('CRC8_E2EProfile1');
  Mux2 : Mux  Inputs=3
  CRC8_E2EResult : Outport
  wires:
  Mux2/1 -> CRC8_E2EProfile1/1(MsgData)
  CAN_E2E_ID1/1 -> Mux2/1
  CAN_E2E_ID2/1 -> Mux2/2
  Byte1/1 -> Mux2/3
  CRC8_E2EProfile1/1(CRCout) -> CRC8_E2EResult/1

== system halout/HAL_OUT/CAN3/FD3_VCU2_toNIDEC_0x154/CRC8_IfAction_Tx/If Action Subsystem ==
  Byte1 : Inport
  Action Port : ActionPort
  CRC8_Caculation : Subsystem
      mask help: MeasumentTrigerEvent
      mask Display: fprintf('CRC8');
  CRC8_Result : Outport
  wires:
  CRC8_Caculation/1(CRCout) -> CRC8_Result/1
  Byte1/1 -> CRC8_Caculation/1(MsgData)

== system halout/HAL_OUT/CAN3/FD3_VCU2_toNIDEC_0x154/CRC8_IfAction_Tx/If Action Subsystem1 ==
  CAN_E2E_ID1 : Inport
  CAN_E2E_ID2 : Inport  Port=2
  Byte1 : Inport  Port=3
  Action Port : ActionPort
  CRC8_E2EProfile1 : Subsystem
      mask help: MeasumentTrigerEvent
      mask Display: fprintf('CRC8_E2EProfile1');
  Mux2 : Mux  Inputs=3
  CRC8_E2EResult : Outport
  wires:
  Mux2/1 -> CRC8_E2EProfile1/1(MsgData)
  CAN_E2E_ID1/1 -> Mux2/1
  CAN_E2E_ID2/1 -> Mux2/2
  Byte1/1 -> Mux2/3
  CRC8_E2EProfile1/1(CRCout) -> CRC8_E2EResult/1

== system halout/HAL_OUT/CAN4/FD4_CE100_0_0x116/CRC8_IfAction_Tx/If Action Subsystem ==
  Byte1 : Inport
  Action Port : ActionPort
  CRC8_Caculation : Subsystem
      mask help: MeasumentTrigerEvent
      mask Display: fprintf('CRC8');
  CRC8_Result : Outport
  wires:
  CRC8_Caculation/1(CRCout) -> CRC8_Result/1
  Byte1/1 -> CRC8_Caculation/1(MsgData)

== system halout/HAL_OUT/CAN4/FD4_CE100_0_0x116/CRC8_IfAction_Tx/If Action Subsystem1 ==
  CAN_E2E_ID1 : Inport
  CAN_E2E_ID2 : Inport  Port=2
  Byte1 : Inport  Port=3
  Action Port : ActionPort
  CRC8_E2EProfile1 : Subsystem
      mask help: MeasumentTrigerEvent
      mask Display: fprintf('CRC8_E2EProfile1');
  Mux2 : Mux  Inputs=3
  CRC8_E2EResult : Outport
  wires:
  Mux2/1 -> CRC8_E2EProfile1/1(MsgData)
  CAN_E2E_ID1/1 -> Mux2/1
  CAN_E2E_ID2/1 -> Mux2/2
  Byte1/1 -> Mux2/3
  CRC8_E2EProfile1/1(CRCout) -> CRC8_E2EResult/1

== system halout/HAL_OUT/CAN6/FD6_APS3_0x238/CRC8_IfAction_Tx/If Action Subsystem ==
  Byte1 : Inport
  Action Port : ActionPort
  CRC8_Caculation : Subsystem
      mask help: MeasumentTrigerEvent
      mask Display: fprintf('CRC8');
  CRC8_Result : Outport
  wires:
  CRC8_Caculation/1(CRCout) -> CRC8_Result/1
  Byte1/1 -> CRC8_Caculation/1(MsgData)

== system halout/HAL_OUT/CAN6/FD6_APS3_0x238/CRC8_IfAction_Tx/If Action Subsystem1 ==
  CAN_E2E_ID1 : Inport
  CAN_E2E_ID2 : Inport  Port=2
  Byte1 : Inport  Port=3
  Action Port : ActionPort
  CRC8_E2EProfile1 : Subsystem
      mask help: MeasumentTrigerEvent
      mask Display: fprintf('CRC8_E2EProfile1');
  Mux2 : Mux  Inputs=3
  CRC8_E2EResult : Outport
  wires:
  Mux2/1 -> CRC8_E2EProfile1/1(MsgData)
  CAN_E2E_ID1/1 -> Mux2/1
  CAN_E2E_ID2/1 -> Mux2/2
  Byte1/1 -> Mux2/3
  CRC8_E2EProfile1/1(CRCout) -> CRC8_E2EResult/1

== system halout/HAL_OUT/CAN6/FD6_VCU2_0x154/CRC8_IfAction_Tx/If Action Subsystem ==
  Byte1 : Inport
  Action Port : ActionPort
  CRC8_Caculation : Subsystem
      mask help: MeasumentTrigerEvent
      mask Display: fprintf('CRC8');
  CRC8_Result : Outport
  wires:
  CRC8_Caculation/1(CRCout) -> CRC8_Result/1
  Byte1/1 -> CRC8_Caculation/1(MsgData)

== system halout/HAL_OUT/CAN6/FD6_VCU2_0x154/CRC8_IfAction_Tx/If Action Subsystem1 ==
  CAN_E2E_ID1 : Inport
  CAN_E2E_ID2 : Inport  Port=2
  Byte1 : Inport  Port=3
  Action Port : ActionPort
  CRC8_E2EProfile1 : Subsystem
      mask help: MeasumentTrigerEvent
      mask Display: fprintf('CRC8_E2EProfile1');
  Mux2 : Mux  Inputs=3
  CRC8_E2EResult : Outport
  wires:
  Mux2/1 -> CRC8_E2EProfile1/1(MsgData)
  CAN_E2E_ID1/1 -> Mux2/1
  CAN_E2E_ID2/1 -> Mux2/2
  Byte1/1 -> Mux2/3
  CRC8_E2EProfile1/1(CRCout) -> CRC8_E2EResult/1

== system halout/HAL_OUT/CAN1/FD1_APS3_0x238/CRC8_IfAction_Tx/If Action Subsystem/CRC8_Caculation ==
  MsgData : Inport
  Data Type Conversion3 : DataTypeConversion  OutDataTypeStr=uint8
  Data Type Conversion4 : DataTypeConversion  OutDataTypeStr=uint8
  MATLAB Function : MATLAB Function  TreatAsAtomicUnit=on
  CRCout : Outport
  wires:
  Data Type Conversion4/1 -> CRCout/1
  MATLAB Function/1(CRC_Out) -> Data Type Conversion4/1
  Data Type Conversion3/1 -> MATLAB Function/1(msg_raw)
  MsgData/1 -> Data Type Conversion3/1

== system halout/HAL_OUT/CAN1/FD1_APS3_0x238/CRC8_IfAction_Tx/If Action Subsystem1/CRC8_E2EProfile1 ==
  MsgData : Inport
  Data Type Conversion3 : DataTypeConversion  OutDataTypeStr=uint8
  Data Type Conversion4 : DataTypeConversion  OutDataTypeStr=uint8
  MATLAB Function : MATLAB Function  TreatAsAtomicUnit=on
  CRCout : Outport
  wires:
  MsgData/1 -> Data Type Conversion3/1
  Data Type Conversion3/1 -> MATLAB Function/1(msg_raw)
  MATLAB Function/1(CRC_Out) -> Data Type Conversion4/1
  Data Type Conversion4/1 -> CRCout/1

== system halout/HAL_OUT/CAN1/FD1_VCU2_0x154/CRC8_IfAction_Tx/If Action Subsystem/CRC8_Caculation ==
  MsgData : Inport
  Data Type Conversion3 : DataTypeConversion  OutDataTypeStr=uint8
  Data Type Conversion4 : DataTypeConversion  OutDataTypeStr=uint8
  MATLAB Function : MATLAB Function  TreatAsAtomicUnit=on
  CRCout : Outport
  wires:
  Data Type Conversion4/1 -> CRCout/1
  MATLAB Function/1(CRC_Out) -> Data Type Conversion4/1
  Data Type Conversion3/1 -> MATLAB Function/1(msg_raw)
  MsgData/1 -> Data Type Conversion3/1

== system halout/HAL_OUT/CAN1/FD1_VCU2_0x154/CRC8_IfAction_Tx/If Action Subsystem1/CRC8_E2EProfile1 ==
  MsgData : Inport
  Data Type Conversion3 : DataTypeConversion  OutDataTypeStr=uint8
  Data Type Conversion4 : DataTypeConversion  OutDataTypeStr=uint8
  MATLAB Function : MATLAB Function  TreatAsAtomicUnit=on
  CRCout : Outport
  wires:
  MsgData/1 -> Data Type Conversion3/1
  Data Type Conversion3/1 -> MATLAB Function/1(msg_raw)
  MATLAB Function/1(CRC_Out) -> Data Type Conversion4/1
  Data Type Conversion4/1 -> CRCout/1

== system halout/HAL_OUT/CAN1/FD1_VCU3_0x159/CRC8_IfAction_Tx/If Action Subsystem/CRC8_Caculation ==
  MsgData : Inport
  Data Type Conversion3 : DataTypeConversion  OutDataTypeStr=uint8
  Data Type Conversion4 : DataTypeConversion  OutDataTypeStr=uint8
  MATLAB Function : MATLAB Function  TreatAsAtomicUnit=on
  CRCout : Outport
  wires:
  Data Type Conversion4/1 -> CRCout/1
  MATLAB Function/1(CRC_Out) -> Data Type Conversion4/1
  Data Type Conversion3/1 -> MATLAB Function/1(msg_raw)
  MsgData/1 -> Data Type Conversion3/1

== system halout/HAL_OUT/CAN1/FD1_VCU3_0x159/CRC8_IfAction_Tx/If Action Subsystem1/CRC8_E2EProfile1 ==
  MsgData : Inport
  Data Type Conversion3 : DataTypeConversion  OutDataTypeStr=uint8
  Data Type Conversion4 : DataTypeConversion  OutDataTypeStr=uint8
  MATLAB Function : MATLAB Function  TreatAsAtomicUnit=on
  CRCout : Outport
  wires:
  MsgData/1 -> Data Type Conversion3/1
  Data Type Conversion3/1 -> MATLAB Function/1(msg_raw)
  MATLAB Function/1(CRC_Out) -> Data Type Conversion4/1
  Data Type Conversion4/1 -> CRCout/1

== system halout/HAL_OUT/CAN1/VMC_FCM1_0x172/CRC8_IfAction_Tx/If Action Subsystem/CRC8_Caculation ==
  MsgData : Inport
  Data Type Conversion3 : DataTypeConversion  OutDataTypeStr=uint8
  Data Type Conversion4 : DataTypeConversion  OutDataTypeStr=uint8
  MATLAB Function : MATLAB Function  TreatAsAtomicUnit=on
  CRCout : Outport
  wires:
  Data Type Conversion4/1 -> CRCout/1
  MATLAB Function/1(CRC_Out) -> Data Type Conversion4/1
  Data Type Conversion3/1 -> MATLAB Function/1(msg_raw)
  MsgData/1 -> Data Type Conversion3/1

== system halout/HAL_OUT/CAN1/VMC_FCM1_0x172/CRC8_IfAction_Tx/If Action Subsystem1/CRC8_E2EProfile1 ==
  MsgData : Inport
  Data Type Conversion3 : DataTypeConversion  OutDataTypeStr=uint8
  Data Type Conversion4 : DataTypeConversion  OutDataTypeStr=uint8
  MATLAB Function : MATLAB Function  TreatAsAtomicUnit=on
  CRCout : Outport
  wires:
  MsgData/1 -> Data Type Conversion3/1
  Data Type Conversion3/1 -> MATLAB Function/1(msg_raw)
  MATLAB Function/1(CRC_Out) -> Data Type Conversion4/1
  Data Type Conversion4/1 -> CRCout/1

== system halout/HAL_OUT/CAN3/FD3_VCU2_0x153/CRC8_IfAction_Tx/If Action Subsystem/CRC8_Caculation ==
  MsgData : Inport
  Data Type Conversion3 : DataTypeConversion  OutDataTypeStr=uint8
  Data Type Conversion4 : DataTypeConversion  OutDataTypeStr=uint8
  MATLAB Function : MATLAB Function  TreatAsAtomicUnit=on
  CRCout : Outport
  wires:
  Data Type Conversion4/1 -> CRCout/1
  MATLAB Function/1(CRC_Out) -> Data Type Conversion4/1
  Data Type Conversion3/1 -> MATLAB Function/1(msg_raw)
  MsgData/1 -> Data Type Conversion3/1

== system halout/HAL_OUT/CAN3/FD3_VCU2_0x153/CRC8_IfAction_Tx/If Action Subsystem1/CRC8_E2EProfile1 ==
  MsgData : Inport
  Data Type Conversion3 : DataTypeConversion  OutDataTypeStr=uint8
  Data Type Conversion4 : DataTypeConversion  OutDataTypeStr=uint8
  MATLAB Function : MATLAB Function  TreatAsAtomicUnit=on
  CRCout : Outport
  wires:
  MsgData/1 -> Data Type Conversion3/1
  Data Type Conversion3/1 -> MATLAB Function/1(msg_raw)
  MATLAB Function/1(CRC_Out) -> Data Type Conversion4/1
  Data Type Conversion4/1 -> CRCout/1

== system halout/HAL_OUT/CAN3/FD3_VCU2_toNIDEC_0x154/CRC8_IfAction_Tx/If Action Subsystem/CRC8_Caculation ==
  MsgData : Inport
  Data Type Conversion3 : DataTypeConversion  OutDataTypeStr=uint8
  Data Type Conversion4 : DataTypeConversion  OutDataTypeStr=uint8
  MATLAB Function : MATLAB Function  TreatAsAtomicUnit=on
  CRCout : Outport
  wires:
  Data Type Conversion4/1 -> CRCout/1
  MATLAB Function/1(CRC_Out) -> Data Type Conversion4/1
  Data Type Conversion3/1 -> MATLAB Function/1(msg_raw)
  MsgData/1 -> Data Type Conversion3/1

== system halout/HAL_OUT/CAN3/FD3_VCU2_toNIDEC_0x154/CRC8_IfAction_Tx/If Action Subsystem1/CRC8_E2EProfile1 ==
  MsgData : Inport
  Data Type Conversion3 : DataTypeConversion  OutDataTypeStr=uint8
  Data Type Conversion4 : DataTypeConversion  OutDataTypeStr=uint8
  MATLAB Function : MATLAB Function  TreatAsAtomicUnit=on
  CRCout : Outport
  wires:
  MsgData/1 -> Data Type Conversion3/1
  Data Type Conversion3/1 -> MATLAB Function/1(msg_raw)
  MATLAB Function/1(CRC_Out) -> Data Type Conversion4/1
  Data Type Conversion4/1 -> CRCout/1

== system halout/HAL_OUT/CAN4/FD4_CE100_0_0x116/CRC8_IfAction_Tx/If Action Subsystem/CRC8_Caculation ==
  MsgData : Inport
  Data Type Conversion3 : DataTypeConversion  OutDataTypeStr=uint8
  Data Type Conversion4 : DataTypeConversion  OutDataTypeStr=uint8
  MATLAB Function : MATLAB Function  TreatAsAtomicUnit=on
  CRCout : Outport
  wires:
  Data Type Conversion4/1 -> CRCout/1
  MATLAB Function/1(CRC_Out) -> Data Type Conversion4/1
  Data Type Conversion3/1 -> MATLAB Function/1(msg_raw)
  MsgData/1 -> Data Type Conversion3/1

== system halout/HAL_OUT/CAN4/FD4_CE100_0_0x116/CRC8_IfAction_Tx/If Action Subsystem1/CRC8_E2EProfile1 ==
  MsgData : Inport
  Data Type Conversion3 : DataTypeConversion  OutDataTypeStr=uint8
  Data Type Conversion4 : DataTypeConversion  OutDataTypeStr=uint8
  MATLAB Function : MATLAB Function  TreatAsAtomicUnit=on
  CRCout : Outport
  wires:
  MsgData/1 -> Data Type Conversion3/1
  Data Type Conversion3/1 -> MATLAB Function/1(msg_raw)
  MATLAB Function/1(CRC_Out) -> Data Type Conversion4/1
  Data Type Conversion4/1 -> CRCout/1

== system halout/HAL_OUT/CAN6/FD6_APS3_0x238/CRC8_IfAction_Tx/If Action Subsystem/CRC8_Caculation ==
  MsgData : Inport
  Data Type Conversion3 : DataTypeConversion  OutDataTypeStr=uint8
  Data Type Conversion4 : DataTypeConversion  OutDataTypeStr=uint8
  MATLAB Function : MATLAB Function  TreatAsAtomicUnit=on
  CRCout : Outport
  wires:
  Data Type Conversion4/1 -> CRCout/1
  MATLAB Function/1(CRC_Out) -> Data Type Conversion4/1
  Data Type Conversion3/1 -> MATLAB Function/1(msg_raw)
  MsgData/1 -> Data Type Conversion3/1

== system halout/HAL_OUT/CAN6/FD6_APS3_0x238/CRC8_IfAction_Tx/If Action Subsystem1/CRC8_E2EProfile1 ==
  MsgData : Inport
  Data Type Conversion3 : DataTypeConversion  OutDataTypeStr=uint8
  Data Type Conversion4 : DataTypeConversion  OutDataTypeStr=uint8
  MATLAB Function : MATLAB Function  TreatAsAtomicUnit=on
  CRCout : Outport
  wires:
  MsgData/1 -> Data Type Conversion3/1
  Data Type Conversion3/1 -> MATLAB Function/1(msg_raw)
  MATLAB Function/1(CRC_Out) -> Data Type Conversion4/1
  Data Type Conversion4/1 -> CRCout/1

== system halout/HAL_OUT/CAN6/FD6_VCU2_0x154/CRC8_IfAction_Tx/If Action Subsystem/CRC8_Caculation ==
  MsgData : Inport
  Data Type Conversion3 : DataTypeConversion  OutDataTypeStr=uint8
  Data Type Conversion4 : DataTypeConversion  OutDataTypeStr=uint8
  MATLAB Function : MATLAB Function  TreatAsAtomicUnit=on
  CRCout : Outport
  wires:
  Data Type Conversion4/1 -> CRCout/1
  MATLAB Function/1(CRC_Out) -> Data Type Conversion4/1
  Data Type Conversion3/1 -> MATLAB Function/1(msg_raw)
  MsgData/1 -> Data Type Conversion3/1

== system halout/HAL_OUT/CAN6/FD6_VCU2_0x154/CRC8_IfAction_Tx/If Action Subsystem1/CRC8_E2EProfile1 ==
  MsgData : Inport
  Data Type Conversion3 : DataTypeConversion  OutDataTypeStr=uint8
  Data Type Conversion4 : DataTypeConversion  OutDataTypeStr=uint8
  MATLAB Function : MATLAB Function  TreatAsAtomicUnit=on
  CRCout : Outport
  wires:
  MsgData/1 -> Data Type Conversion3/1
  Data Type Conversion3/1 -> MATLAB Function/1(msg_raw)
  MATLAB Function/1(CRC_Out) -> Data Type Conversion4/1
  Data Type Conversion4/1 -> CRCout/1

== stateflow chart halout/HAL_OUT/CAN1/FD1_VCU2_Tx/Chart ==
  state TrigCounter
    en:
    counter = 0;
    counter++;
    (default) -> (junction 5)
    TrigCounter -> (junction 5) : {
        | counter++;
        | }
    (junction 5) -> (junction 6) [order 1] : [TxReq && (counter %% CycleCnt) == 0]
    (junction 5) -> (junction 7) [order 2]
    (junction 6) -> (junction 8) : {
        | TxTrigger;
        | counter = 0;
        | }
    (junction 8) -> (junction 7)
    (junction 7) -> (junction 34)
    (junction 34) -> (junction 33) [order 1] : [ !TxReq]
    (junction 34) -> (junction 35) [order 2]
    (junction 33) -> (junction 36) : {
        | counter = 0;
        | }
    (junction 36) -> (junction 35)
    (junction 35) -> (junction 44)
  data: TxReq input; CycleCnt input; counter local uint16
  events: TxTrigger output FUNCTION_CALL_EVENT

== matlab function halout/HAL_OUT/CAN1/FD1_APS3_0x238/CRC8_IfAction_Tx/If Action Subsystem1/CRC8_E2EProfile1/MATLAB Function ==
  data: msg_raw input; CRC_Out output
function CRC_Out= fcn(msg_raw)

divisor = 0x1D;
messageLength = 8;
CRC_raw = uint8(0x00);

for i = 1:length(msg_raw(:,1))

    message = bitxor(CRC_raw,msg_raw(i));

    for k = 1:messageLength
        if bitget(message,8)
            message = bitshift(message,1);
            message = bitxor(message,divisor);
        else
            message = bitshift(message,1);
        end
    end
    CRC_raw = message;

end

CRC_Out = bitxor(CRC_raw,0x00);

== stateflow chart halout/HAL_OUT/CAN1/FD1_APS3_Tx/Chart ==
  state TrigCounter
    en:
    counter = 0;
    counter++;
    (default) -> (junction 5)
    TrigCounter -> (junction 5) : {
        | counter++;
        | }
    (junction 5) -> (junction 6) [order 1] : [TxReq && (counter %% CycleCnt) == 0]
    (junction 5) -> (junction 7) [order 2]
    (junction 6) -> (junction 8) : {
        | TxTrigger;
        | counter = 0;
        | }
    (junction 8) -> (junction 7)
    (junction 7) -> (junction 34)
    (junction 34) -> (junction 33) [order 1] : [ !TxReq]
    (junction 34) -> (junction 35) [order 2]
    (junction 33) -> (junction 36) : {
        | counter = 0;
        | }
    (junction 36) -> (junction 35)
    (junction 35) -> (junction 44)
  data: TxReq input; CycleCnt input; counter local uint16
  events: TxTrigger output FUNCTION_CALL_EVENT

== matlab function halout/HAL_OUT/CAN1/FD1_VCU2_0x154/CRC8_IfAction_Tx/If Action Subsystem/CRC8_Caculation/MATLAB Function ==
  data: msg_raw input; CRC_Out output
function CRC_Out= fcn(msg_raw)

divisor = 0x1D;
messageLength = 8;
CRC_raw = uint8(0xFF);

for i = 1:length(msg_raw(:,1))

    message = bitxor(CRC_raw,msg_raw(i));

    for k = 1:messageLength
        if bitget(message,8)
            message = bitshift(message,1);
            message = bitxor(message,divisor);
        else
            message = bitshift(message,1);
        end
    end
    CRC_raw = message;

end

CRC_Out = bitxor(CRC_raw,0xFF);

== matlab function halout/HAL_OUT/CAN1/FD1_VCU2_0x154/CRC8_IfAction_Tx/If Action Subsystem1/CRC8_E2EProfile1/MATLAB Function ==
  data: msg_raw input; CRC_Out output
function CRC_Out= fcn(msg_raw)

divisor = 0x1D;
messageLength = 8;
CRC_raw = uint8(0x00);

for i = 1:length(msg_raw(:,1))

    message = bitxor(CRC_raw,msg_raw(i));

    for k = 1:messageLength
        if bitget(message,8)
            message = bitshift(message,1);
            message = bitxor(message,divisor);
        else
            message = bitshift(message,1);
        end
    end
    CRC_raw = message;

end

CRC_Out = bitxor(CRC_raw,0x00);

== stateflow chart halout/HAL_OUT/CAN1/FD1_VCU3_Tx/Chart ==
  state TrigCounter
    en:
    counter = 0;
    counter++;
    (default) -> (junction 5)
    TrigCounter -> (junction 5) : {
        | counter++;
        | }
    (junction 5) -> (junction 6) [order 1] : [TxReq && (counter %% CycleCnt) == 0]
    (junction 5) -> (junction 7) [order 2]
    (junction 6) -> (junction 8) : {
        | TxTrigger;
        | counter = 0;
        | }
    (junction 8) -> (junction 7)
    (junction 7) -> (junction 34)
    (junction 34) -> (junction 33) [order 1] : [ !TxReq]
    (junction 34) -> (junction 35) [order 2]
    (junction 33) -> (junction 36) : {
        | counter = 0;
        | }
    (junction 36) -> (junction 35)
    (junction 35) -> (junction 44)
  data: TxReq input; CycleCnt input; counter local uint16
  events: TxTrigger output FUNCTION_CALL_EVENT

== matlab function halout/HAL_OUT/CAN1/FD1_VCU3_0x159/CRC8_IfAction_Tx/If Action Subsystem/CRC8_Caculation/MATLAB Function ==
  data: msg_raw input; CRC_Out output
function CRC_Out= fcn(msg_raw)

divisor = 0x1D;
messageLength = 8;
CRC_raw = uint8(0xFF);

for i = 1:length(msg_raw(:,1))

    message = bitxor(CRC_raw,msg_raw(i));

    for k = 1:messageLength
        if bitget(message,8)
            message = bitshift(message,1);
            message = bitxor(message,divisor);
        else
            message = bitshift(message,1);
        end
    end
    CRC_raw = message;

end

CRC_Out = bitxor(CRC_raw,0xFF);

== matlab function halout/HAL_OUT/CAN1/FD1_VCU3_0x159/CRC8_IfAction_Tx/If Action Subsystem1/CRC8_E2EProfile1/MATLAB Function ==
  data: msg_raw input; CRC_Out output
function CRC_Out= fcn(msg_raw)

divisor = 0x1D;
messageLength = 8;
CRC_raw = uint8(0x00);

for i = 1:length(msg_raw(:,1))

    message = bitxor(CRC_raw,msg_raw(i));

    for k = 1:messageLength
        if bitget(message,8)
            message = bitshift(message,1);
            message = bitxor(message,divisor);
        else
            message = bitshift(message,1);
        end
    end
    CRC_raw = message;

end

CRC_Out = bitxor(CRC_raw,0x00);

== stateflow chart halout/HAL_OUT/CAN1/VMC_FCM1_Tx/Chart ==
  state TrigCounter
    en:
    counter = 0;
    counter++;
    (default) -> (junction 5)
    TrigCounter -> (junction 5) : {
        | counter++;
        | }
    (junction 5) -> (junction 6) [order 1] : [TxReq && (counter %% CycleCnt) == 0]
    (junction 5) -> (junction 7) [order 2]
    (junction 6) -> (junction 8) : {
        | TxTrigger;
        | counter = 0;
        | }
    (junction 8) -> (junction 7)
    (junction 7) -> (junction 34)
    (junction 34) -> (junction 33) [order 1] : [ !TxReq]
    (junction 34) -> (junction 35) [order 2]
    (junction 33) -> (junction 36) : {
        | counter = 0;
        | }
    (junction 36) -> (junction 35)
    (junction 35) -> (junction 44)
  data: TxReq input; CycleCnt input; counter local uint16
  events: TxTrigger output FUNCTION_CALL_EVENT
